simulink model "gekopelde_pendulum"  (R2018b)
settings: Solver=VariableStepAuto  StartTime=0.0  StopTime=10.0  RelTol=1e-3
values from neighbouring files (symbols this model uses):
  K = lqr(A,B,Q,R)    [pendulum_version1.m]
  Ts = 1/200    (= 0.005)    [pendulum_version1.m]
undefined symbols (not defined in the file or in its folder): National_Instruments, omega_c, PCI
libraries: sldrtlib x2, simulink_extras x2
settings Model: Creator=paul-emileverleye  LastModifiedBy=paul-emileverleye

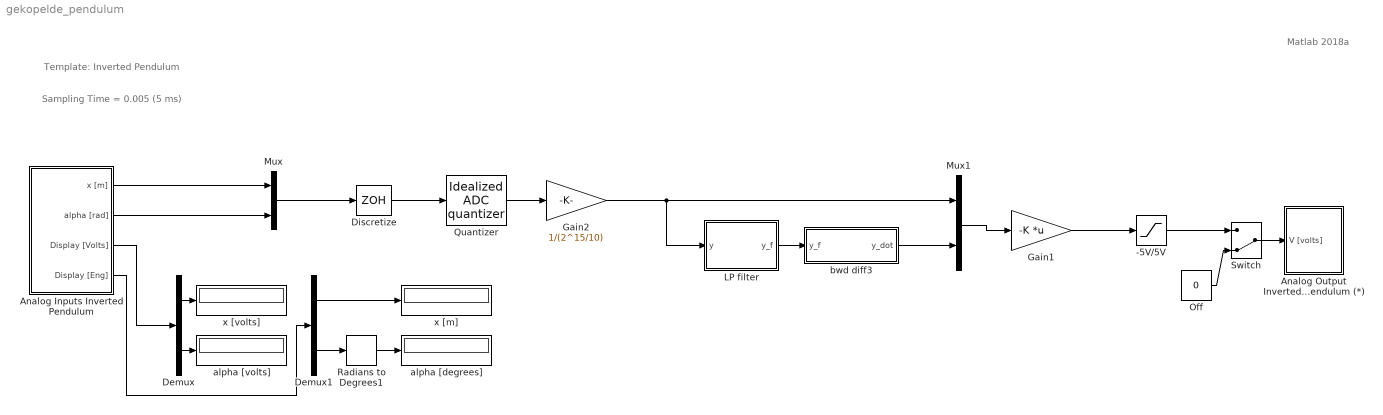
== system gekopelde_pendulum ==
  note: Sampling Time = 0.005 (5 ms)
  note: Template: Inverted Pendulum
  note: Matlab 2018a
  -5V/5V : Saturate  UpperLimit=5  LowerLimit=-5
  Analog Inputs Inverted Pendulum : Subsystem  mask(Analog Inputs. Inverted Pendulum){v2m=0.1033, offset_x=0, v2r=0.2482, offset_alfa=0.17}
      mask prompts: v2m "F_x = Convertion factor from Volts to Meters:"; offset_x "Off_x = Offset for the Cart Position [Volts] :"; v2r "F_alpha = Convertion Factor from Volts to Radians :"; offset_alfa "Off_alpha = Offset for the angle of the rob [Volts] :"
      mask help:
      | Remember:
      |    Cart Position (x)           => channel ACH0
      |    Angle of the rod (alpha) => channel ACH1
      |
      |   Cart Position [m] = F_x * ( Cart Position [v] + off_x )
      |   Angle of the rod [rad] = F_alpha * ( Angle of the rod [v] + off_alpha )
  Analog Output Inverted Pendulum (*) : Subsystem  mask(Analog Output - Inverted Pendulum){}
      mask help:
      | Remember
      |    AO 0 => Power Amplifier + Motor
  Demux : Demux  Outputs=2
  Demux1 : Demux  Outputs=2
  Discretize : ZeroOrderHold  SampleTime=1/200
  Gain1 : Gain  Gain=-K  Multiplication=Matrix(K*u)
  Gain2 : Gain  Gain=1/(2^15/10)
  LP filter : Subsystem
  Mux : Mux  Inputs=2
  Mux1 : Mux  Inputs=2
  Off : Constant  Value=0
  Quantizer : simulink_extras/Additional Discrete/Idealized ADC quantizer  NumberOfConverterBits=16  Vmin=-10  Vmax=10  OutputDataType=double  OutputNegativeValues=on
      settings: SourceProductName=Simulink
  Radians to Degrees1 : simulink_extras/Transformations/Radians to Degrees
  "Switch  " : ManualSwitch  CurrentSetting=0
  alpha [degrees] : Display
  alpha [volts] : Display
  bwd diff3 : Subsystem
  x [m] : Display
  x [volts] : Display
  wires:
  Off/1 -> "Switch  "/2
  Demux1/2 -> Radians to Degrees1/1
  Radians to Degrees1/1 -> alpha [degrees]/1
  Analog Inputs Inverted Pendulum/4(Display [Eng]) -> Demux1/1
  Demux/1 -> x [volts]/1
  Demux/2 -> alpha [volts]/1
  Demux1/1 -> x [m]/1
  "Switch  "/1 -> Analog Output Inverted Pendulum (*)/1(V [volts])
  Analog Inputs Inverted Pendulum/3(Display [Volts]) -> Demux/1
  Quantizer/1 -> Gain2/1
  Analog Inputs Inverted Pendulum/1(x [m]) -> Mux/1
  Analog Inputs Inverted Pendulum/2(alpha [rad]) -> Mux/2
  Mux/1 -> Discretize/1
  LP filter/1(y_f) -> bwd diff3/1(y_f)
  Gain2/1 -> LP filter/1(y), Mux1/1
  bwd diff3/1(y_dot) -> Mux1/2
  -5V/5V/1 -> "Switch  "/1
  Gain1/1 -> -5V/5V/1
  Mux1/1 -> Gain1/1
  Discretize/1 -> Quantizer/1

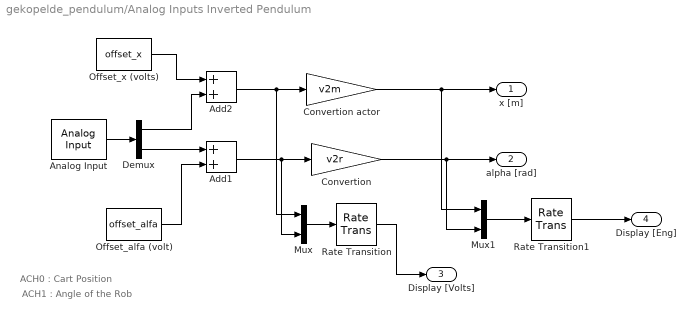
== system gekopelde_pendulum/Analog Inputs Inverted Pendulum ==
  note: ACH0 : Cart Position
  note: ACH1 : Angle of the Rob
  Add1 : Sum
  Add2 : Sum
  Analog Input : sldrtlib/Analog Input  SampleTime=0.005  MaxMissedTicks=10  ShowMissedTicks=off  YieldWhenWaiting=off  DrvName=National_Instruments/PCI-6014  DrvAddress=4294967295  DrvOptions=[1 0 0 0 0 0]  Channels=[1 2]  RangeMode=1  VoltRange=1  DataType=1
      settings: AttributesFormatString=National Instruments\nPCI-6014 [auto]  SourceProductName=Simulink Desktop Real-Time
  "Convertion " : Gain  Gain=v2r
  Convertion actor : Gain  Gain=v2m
  Demux : Demux  Outputs=2
  Mux : Mux  Inputs=2
  Mux1 : Mux  Inputs=2
  Offset_alfa (volt) : Constant  Value=offset_alfa
  Offset_x (volts) : Constant  Value=offset_x
  Rate Transition : RateTransition  OutPortSampleTime=0.25
  Rate Transition1 : RateTransition  OutPortSampleTime=0.25
  x [m] : Outport
  alpha [rad] : Outport  Port=2
  Display [Volts] : Outport  Port=3
  Display [Eng] : Outport  Port=4
  wires:
  Analog Input/1 -> Demux/1
  Demux/1 -> Add2/2
  Add2/1 -> Convertion actor/1, Mux/1
  Offset_x (volts)/1 -> Add2/1
  Convertion actor/1 -> x [m]/1, Mux1/1
  Demux/2 -> Add1/1
  Offset_alfa (volt)/1 -> Add1/2
  Add1/1 -> "Convertion "/1, Mux/2
  "Convertion "/1 -> alpha [rad]/1, Mux1/2
  Mux/1 -> Rate Transition/1
  Rate Transition/1 -> Display [Volts]/1
  Mux1/1 -> Rate Transition1/1
  Rate Transition1/1 -> Display [Eng]/1

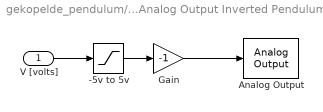
== system gekopelde_pendulum/Analog Output Inverted Pendulum (*) ==
  V [volts] : Inport
  -5v to 5v : Saturate  UpperLimit=5  LowerLimit=-5
  Analog Output : sldrtlib/Analog Output  SampleTime=0.005  MaxMissedTicks=10  ShowMissedTicks=off  YieldWhenWaiting=off  DrvName=National_Instruments/PCI-6014  DrvAddress=4294967295  DrvOptions=[1 0 0 0 0 0]  Channels=1  RangeMode=1  VoltRange=1  InitialValue=0  FinalValue=0
      settings: AttributesFormatString=National Instruments\nPCI-6014 [auto]  SourceProductName=Simulink Desktop Real-Time
  Gain : Gain  Gain=-1
  wires:
  -5v to 5v/1 -> Gain/1
  V [volts]/1 -> -5v to 5v/1
  Gain/1 -> Analog Output/1

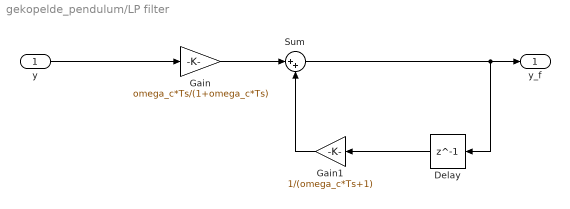
== system gekopelde_pendulum/LP filter ==
  y : Inport
  Delay : Delay  DelayLength=1  InitialCondition=0
  Gain : Gain  Gain=omega_c*Ts/(1+omega_c*Ts)
  Gain1 : Gain  Gain=1/(omega_c*Ts+1)
  Sum : Sum  Inputs=|++
  y_f : Outport
  wires:
  y/1 -> Gain/1
  Gain/1 -> Sum/1
  Delay/1 -> Gain1/1
  Gain1/1 -> Sum/2
  Sum/1 -> Delay/1, y_f/1

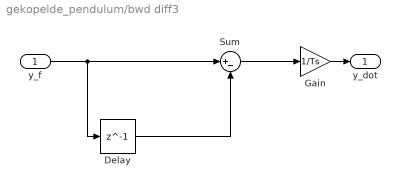
== system gekopelde_pendulum/bwd diff3 ==
  y_f : Inport
  Delay : Delay  DelayLength=1  InitialCondition=0
  Gain : Gain  Gain=1/Ts
  Sum : Sum  Inputs=|+-
  y_dot : Outport
  wires:
  y_f/1 -> Sum/1, Delay/1
  Gain/1 -> y_dot/1
  Delay/1 -> Sum/2
  Sum/1 -> Gain/1
